simulink model "AMR_MotorStartupUnit_23b"  (R2024a)
settings: Solver=FixedStepAuto  StartTime=0.0  StopTime=10.0  FixedStep=1e-3  RelTol=1e-3
settings Model: DataDictionary=configuration_dictionary.sldd  Creator=matlab.cut  LastModifiedBy=matlab.cut
settings SolverCC: ConcurrentTasks=on  PositivePriorityOrder=on
settings OptimizationCC: BlockReduction=off  DefaultParameterBehavior=Inlined  OptimizeBlockIOStorage=off
settings DebuggingCC: TasksWithSamePriorityMsg=none
settings HardwareCC: ProdBitPerLong=64  ProdLongLongMode=on  ProdHWDeviceType=Intel->x86-64 (Linux 64)
settings ModelReferenceCC: ModelReferenceNumInstancesAllowed=Single
settings SFSimCC: MATLABDynamicMemAlloc=off
settings RTWCC: Description=Speedgoat Real-Time Target Machine  SystemTargetFile=speedgoat.tlc  TemplateMakefile=slrealtime_default_tmf  Toolchain=Simulink Real-Time Toolchain  BuildConfiguration=Faster Runs  CodeExecutionProfiling=on  TargetLang=C++  GPUComputeCapability=3.5
settings CodeAppCC: MaxIdLength=127
settings SimulinkRealTimeTargetCC: InstructionSetFMA=off  LogToMDFFile=off

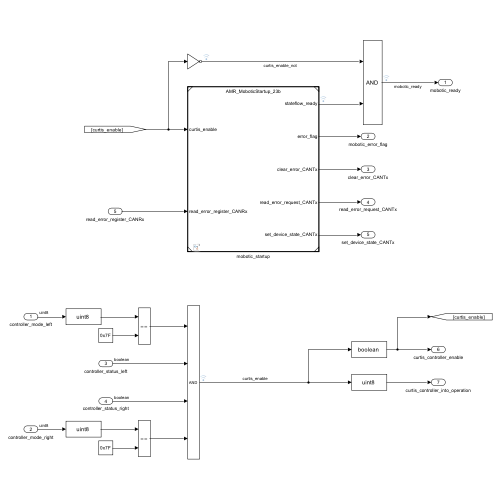
[thumbnail: Simulink's stored preview of the top-level diagram]
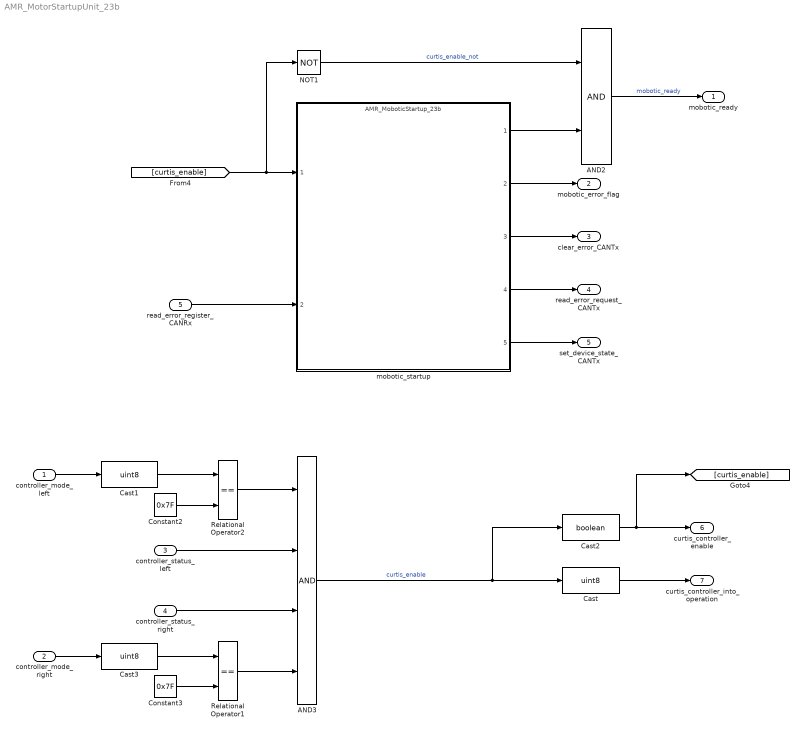
== system AMR_MotorStartupUnit_23b ==
  controller_mode_left : Inport  OutDataTypeStr=uint8
  controller_mode_right : Inport  Port=2  OutDataTypeStr=uint8
  controller_status_left : Inport  Port=3  OutDataTypeStr=boolean
  controller_status_right : Inport  Port=4  OutDataTypeStr=boolean
  read_error_register_CANRx : Inport  Port=5
  AND2 : Logic  AllPortsSameDT=off  OutDataTypeStr=boolean
  AND3 : Logic  Inputs=4  AllPortsSameDT=off  OutDataTypeStr=boolean
  Cast : DataTypeConversion  OutDataTypeStr=uint8  SaturateOnIntegerOverflow=off  RndMeth=Floor
  Cast1 : DataTypeConversion  OutDataTypeStr=uint8  SaturateOnIntegerOverflow=off  RndMeth=Floor
  Cast2 : DataTypeConversion  OutDataTypeStr=boolean  SaturateOnIntegerOverflow=off  RndMeth=Floor
  Cast3 : DataTypeConversion  OutDataTypeStr=uint8  SaturateOnIntegerOverflow=off  RndMeth=Floor
  Constant2 : Constant  Value=0x7F
  Constant3 : Constant  Value=0x7F
  NOT1 : Logic  Operator=NOT  IconShape=distinctive  AllPortsSameDT=off  OutDataTypeStr=boolean
  Relational Operator1 : RelationalOperator  Operator===  OutDataTypeStr=boolean  RndMeth=Simplest  InputSameDT=off
  Relational Operator2 : RelationalOperator  Operator===  OutDataTypeStr=boolean  RndMeth=Simplest  InputSameDT=off
  mobotic_startup : ModelReference  ModelNameDialog=AMR_MoboticStartup_23b.slx  SimulationMode=Normal  ModelReferenceVersion=2.28
  mobotic_ready : Outport
  mobotic_error_flag : Outport  Port=2
  clear_error_CANTx : Outport  Port=3
  read_error_request_CANTx : Outport  Port=4
  set_device_state_CANTx : Outport  Port=5
  curtis_controller_enable : Outport  Port=6
  curtis_controller_into_operation : Outport  Port=7
  wires:
  Constant3/1 -> Relational Operator1/2
  Constant2/1 -> Relational Operator2/2
  AND3/1 -> Cast2/1, Cast/1  "curtis_enable"
  Relational Operator2/1 -> AND3/1
  Relational Operator1/1 -> AND3/4
  NOT1/1 -> AND2/1  "curtis_enable_not"
  [curtis_enable] -> NOT1/1, mobotic_startup/1
  mobotic_startup/1 -> AND2/2
  AND2/1 -> mobotic_ready/1  "mobotic_ready"
  mobotic_startup/2 -> mobotic_error_flag/1
  Cast/1 -> curtis_controller_into_operation/1
  Cast2/1 -> [curtis_enable], curtis_controller_enable/1
  controller_status_left/1 -> AND3/2
  controller_status_right/1 -> AND3/3
  controller_mode_left/1 -> Cast1/1
  controller_mode_right/1 -> Cast3/1
  Cast1/1 -> Relational Operator2/1
  Cast3/1 -> Relational Operator1/1
  mobotic_startup/3 -> clear_error_CANTx/1
  mobotic_startup/4 -> read_error_request_CANTx/1
  mobotic_startup/5 -> set_device_state_CANTx/1
  read_error_register_CANRx/1 -> mobotic_startup/2
